simulink model "Gui"  (R2020b)
settings: Solver=VariableStepAuto  StartTime=0.0  StopTime=inf  RelTol=1e-3
libraries: simulink x7
settings Model: Creator=Axela  LastModifiedBy=MSI PC

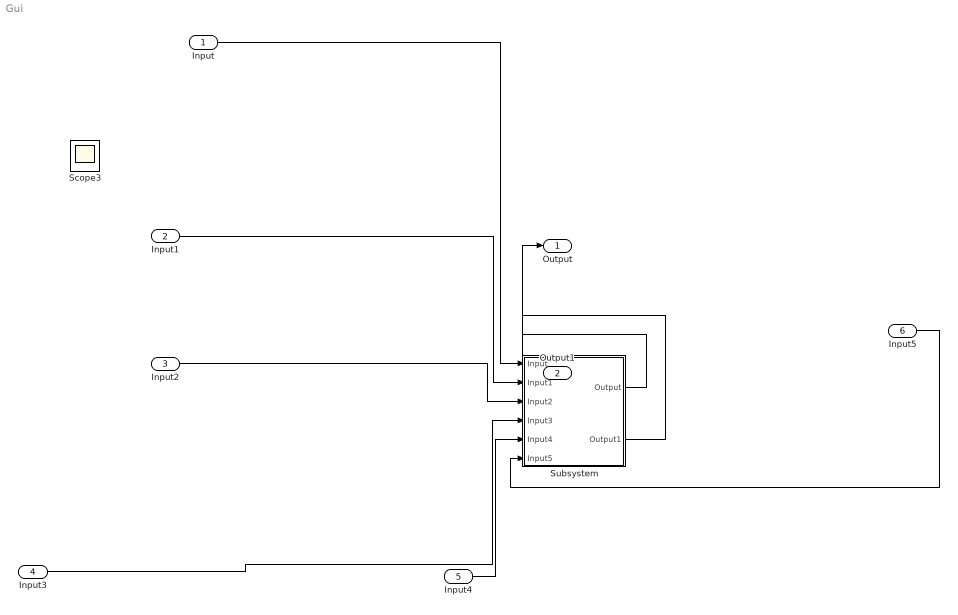
== system Gui ==
  Input : Inport
  Input1 : Inport  Port=2
  Input2 : Inport  Port=3
  Input3 : Inport  Port=4
  Input4 : Inport  Port=5
  Input5 : Inport  Port=6
  Subsystem : Subsystem
  Output : Outport
  Output1 : Outport  Port=2
  Scope3 : Scope
  wires:
  Input/1 -> Subsystem/1(Input)
  Input1/1 -> Subsystem/2(Input1)
  Input2/1 -> Subsystem/3(Input2)
  Input3/1 -> Subsystem/4(Input3)
  Input4/1 -> Subsystem/5(Input4)
  Input5/1 -> Subsystem/6(Input5)
  Subsystem/1(Output) -> Output/1
  Subsystem/2(Output1) -> Output1/1

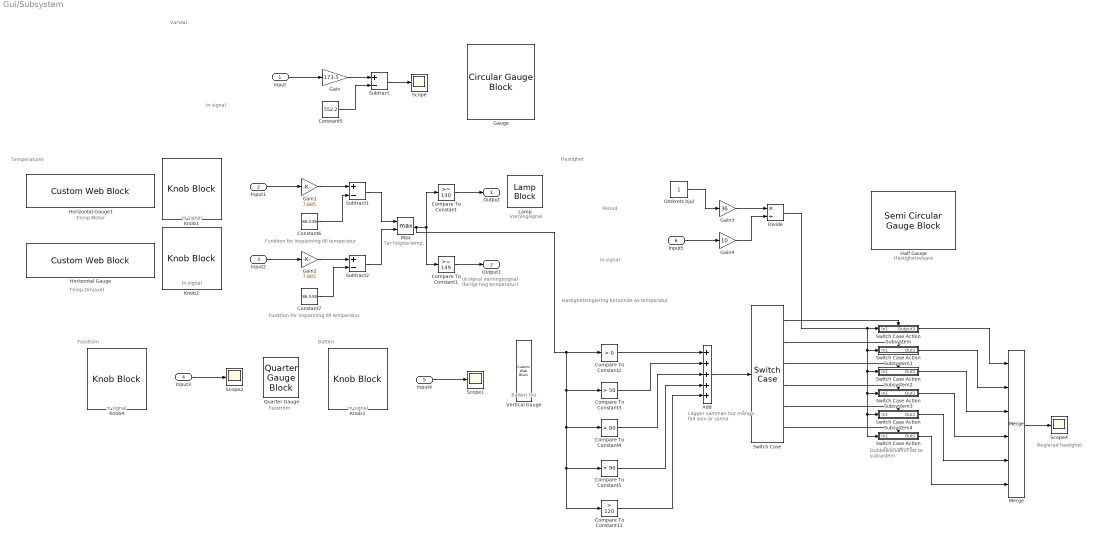
== system Gui/Subsystem ==
  note: in-signal
  note: Tar högsta temp.
  note: Funktion för inspänning till temperatur
  note: Temp.Drivaxel
  note: Temp.Motor
  note: Hastighetsvisare
  note: Reglerad hastighet
  note: Dubbelklicka för att se
      | subsystem
  note: Lägger samman
      | hur många fall
      | som är sanna
  note: Varningsignal
  note: ut-signal varningssignal
      | (farligt hög temperatur)
  note: Fasström
  note: Batteri (%)
  note: in-signal
  note: Hastighetsreglering beroende av temperatur
  note: Batteri
  note: Fasström
  note: Varvtal
  note: Temperaturer
  note: Hastighet
  note: Period
  note: in-signal
  note: in-signal
  note: in-signal
  note: in-signal
  note: Funktion för inspänning till temperatur
  Input : Inport
  Input1 : Inport  Port=2
  Input2 : Inport  Port=3
  Input3 : Inport  Port=4
  Input4 : Inport  Port=5
  Input5 : Inport  Port=6
  Add : Sum  Inputs=+++++
  Compare To Constant : simulink/Logic and Bit Operations/Compare To Constant  relop=>=  const=130  OutDataTypeStr=boolean
  Compare To Constant1 : simulink/Logic and Bit Operations/Compare To Constant  relop=>=  const=149  OutDataTypeStr=boolean
  Compare To Constant11 : simulink/Logic and Bit Operations/Compare To Constant  relop=>  const=120  OutDataTypeStr=boolean
  Compare To Constant2 : simulink/Logic and Bit Operations/Compare To Constant  relop=>  const=0  OutDataTypeStr=boolean
  Compare To Constant3 : simulink/Logic and Bit Operations/Compare To Constant  relop=>  const=50  OutDataTypeStr=boolean
  Compare To Constant4 : simulink/Logic and Bit Operations/Compare To Constant  relop=>  const=80  OutDataTypeStr=boolean
  Compare To Constant5 : simulink/Logic and Bit Operations/Compare To Constant  relop=>  const=90  OutDataTypeStr=boolean
  Constant5 : Constant  Value=552.2
  Constant6 : Constant  Value=86.538
  Constant7 : Constant  Value=86.538
  Divide : Product  Inputs=*/
  Gain : Gain  Gain=173.5
  Gain1 : Gain  Gain=7.885
  Gain2 : Gain  Gain=7.885
  Gain3 : Gain  Gain=36
  Gain4 : Gain  Gain=10
  Gauge : CircularGaugeBlock  LabelPosition=Hide
  Half Gauge : SemiCircularGaugeBlock  LabelPosition=Hide
  Horizontal Gauge : CustomWebBlock  LabelPosition=Hide  ShowInitialText=on  Configuration="{\"components\":[{\"name\":\"LinearScaleComponent\",\"settings\":{\"bounds\":{\"max\":100,\"min\":0,\"tickInterval\":\"auto\"},\"internalTickHeightScaleFactor\":0.5,\"labelColor\":[250,245,199],\"labelFont\":{\"font\":\"Arial\",\"fontSize\":12},\"labelTransparency\":1,\"needleImage\":{\"size\":[21,75],\"src\":\"data:image\\/svg+xml;base64,PHN2ZyB4bWxucz0iaHR0cDovL3d3dy53My5vcmcvMjAwMC9zdmciIHhtbG5zOnhsaW5rPSJodHRwOi8vd3d3LnczLm9yZy8xOTk5L3hsaW5rIiB2aWV3Qm94PSIwIDAgMjEgNzUiPjxkZWZzPjxzdHlsZT4uY2xzLTF7ZmlsbDpub25lO30uY2xzLTJ7aXNvbGF0aW9uOmlzb2xhdGU7fS5jbHMtM3tjbGlwLXBhdGg6dXJsKCNjbGlwLXBhdGgpO30uY2xzLTR7b3BhY2l0eTowLjM7bWl4LWJsZW5kLW1vZGU6bXVsdGlwbHk7fS5jbHMtNXtmaWxsOiNlYjI2Mjk7fTwvc3R5bGU+PGNsaXBQYXRoIGlkPSJjbGlwLXBhdGgiIHRyYW5zZm9y ...(+1928 chars)\",\"srcOrientation\":\"horizontal\"},\"needleOffset\":[0,0.01094391244870041],\"needleSize\":{\"height\":0.7589285714285714,\"width\":0.11960078534031414},\"position\":[0.06986607142857143,0.01995798319327731,0.9641544117647058,0.8],\"scaleColors\":[],\"scaleColorsSize\":0.2,\"showLabels\":1,\"showMinorTicks\":0,\"showSpanLine\":1,\"showTicks\":1,\"tickColor\":[250,245,200],\"tickTransparency\":1,\"valueBarColor\":[23,89,176],\"valueBarOffset\":0,\"valueBarSize\":0.23,\"valueBarTransparency\":1}},{\"name\":\"BackgroundImageComponent\",\"settings\":{\"image\":{\"size\":[380,101],\"src\":\"data:image\\/svg+xml;base64,PHN2ZyB4bWxucz0iaHR0cDovL3d3dy53My5vcmcvMjAwMC9zdmciIHZpZXdCb3g9IjAgMCAzODAgMTAxIj48ZGVmcz48c3R5bGU+LmNscy0xe2ZpbGw6IzAwMmI0Mjt9LmNscy0ye2ZpbGw6IzQyNzA4Mjt9LmNscy0ze2ZpbGw6IzdjYTBiMjt9PC9zdHlsZT48L2RlZnM+PHRpdGxlPmhvcml6b250YWxfZ2F1Z2VfIGJhY2tncm91bmQ8L3RpdGxlPjxnIGlkPSJMYXllcl8yIiBkYXRhLW5hbWU9IkxheWVyIDIiPjxnIGlkPSJMYXllcl8xLTIiIGRhdGEtbmFtZT0iTGF5ZXIgMSI+PHJlY3QgY2xhc3M9ImNscy0xIiB4PSIxMSIgeT0iMTEiIHdpZHRoPSIzNTgiIGhlaWdodD0iNzkiLz48cGF0aCBjbGFzcz0iY2xzLTIiIGQ9Ik04LDhWOTNIMzcyVjhaTTM2OSw5MEgxMVYxMUgzNjlaIi8+PHBhdGggY2xhc3M9ImNscy0zIiBkPSJNMCwwVjEwMUgzODBWMFpNMzcyLDkzSDhWOEgzNzJaIi8+PC9nPjwvZz48L3N2Zz4=\",\"srcOrientation\":\"horizontal\"},\"position\":[0,0,1,1],\"scaleMode\":\"0\"}},{\"name\":\"ForegroundImageComponent\",\"settings\":{\"image\":{\"size\":[0,0],\"src\":\"default\",\"srcOrientation\":[]},\"isForeground\":1,\"position\":[0,0,1,1],\"scaleMode\":\"0\"}}],\"settings\":{\"BindingType\":\"signal\",\"aspectRatio\":3.7721518987341773,\"fixedAspectRatio\":\"on\",\"orientation\":\"horizontal\"},\"type\":\"LinearGauge\"}"
  Horizontal Gauge1 : CustomWebBlock  LabelPosition=Hide  ShowInitialText=on  Configuration="{\"components\":[{\"name\":\"LinearScaleComponent\",\"settings\":{\"bounds\":{\"max\":100,\"min\":0,\"tickInterval\":\"auto\"},\"internalTickHeightScaleFactor\":0.5,\"labelColor\":[250,245,199],\"labelFont\":{\"font\":\"Arial\",\"fontSize\":12},\"labelTransparency\":1,\"needleImage\":{\"size\":[21,75],\"src\":\"data:image\\/svg+xml;base64,PHN2ZyB4bWxucz0iaHR0cDovL3d3dy53My5vcmcvMjAwMC9zdmciIHhtbG5zOnhsaW5rPSJodHRwOi8vd3d3LnczLm9yZy8xOTk5L3hsaW5rIiB2aWV3Qm94PSIwIDAgMjEgNzUiPjxkZWZzPjxzdHlsZT4uY2xzLTF7ZmlsbDpub25lO30uY2xzLTJ7aXNvbGF0aW9uOmlzb2xhdGU7fS5jbHMtM3tjbGlwLXBhdGg6dXJsKCNjbGlwLXBhdGgpO30uY2xzLTR7b3BhY2l0eTowLjM7bWl4LWJsZW5kLW1vZGU6bXVsdGlwbHk7fS5jbHMtNXtmaWxsOiNlYjI2Mjk7fTwvc3R5bGU+PGNsaXBQYXRoIGlkPSJjbGlwLXBhdGgiIHRyYW5zZm9y ...(+1928 chars)\",\"srcOrientation\":\"horizontal\"},\"needleOffset\":[0,0.01094391244870041],\"needleSize\":{\"height\":0.7589285714285714,\"width\":0.11960078534031414},\"position\":[0.06986607142857143,0.01995798319327731,0.9641544117647058,0.8],\"scaleColors\":[],\"scaleColorsSize\":0.2,\"showLabels\":1,\"showMinorTicks\":0,\"showSpanLine\":1,\"showTicks\":1,\"tickColor\":[250,245,200],\"tickTransparency\":1,\"valueBarColor\":[23,89,176],\"valueBarOffset\":0,\"valueBarSize\":0.23,\"valueBarTransparency\":1}},{\"name\":\"BackgroundImageComponent\",\"settings\":{\"image\":{\"size\":[380,101],\"src\":\"data:image\\/svg+xml;base64,PHN2ZyB4bWxucz0iaHR0cDovL3d3dy53My5vcmcvMjAwMC9zdmciIHZpZXdCb3g9IjAgMCAzODAgMTAxIj48ZGVmcz48c3R5bGU+LmNscy0xe2ZpbGw6IzAwMmI0Mjt9LmNscy0ye2ZpbGw6IzQyNzA4Mjt9LmNscy0ze2ZpbGw6IzdjYTBiMjt9PC9zdHlsZT48L2RlZnM+PHRpdGxlPmhvcml6b250YWxfZ2F1Z2VfIGJhY2tncm91bmQ8L3RpdGxlPjxnIGlkPSJMYXllcl8yIiBkYXRhLW5hbWU9IkxheWVyIDIiPjxnIGlkPSJMYXllcl8xLTIiIGRhdGEtbmFtZT0iTGF5ZXIgMSI+PHJlY3QgY2xhc3M9ImNscy0xIiB4PSIxMSIgeT0iMTEiIHdpZHRoPSIzNTgiIGhlaWdodD0iNzkiLz48cGF0aCBjbGFzcz0iY2xzLTIiIGQ9Ik04LDhWOTNIMzcyVjhaTTM2OSw5MEgxMVYxMUgzNjlaIi8+PHBhdGggY2xhc3M9ImNscy0zIiBkPSJNMCwwVjEwMUgzODBWMFpNMzcyLDkzSDhWOEgzNzJaIi8+PC9nPjwvZz48L3N2Zz4=\",\"srcOrientation\":\"horizontal\"},\"position\":[0,0,1,1],\"scaleMode\":\"0\"}},{\"name\":\"ForegroundImageComponent\",\"settings\":{\"image\":{\"size\":[0,0],\"src\":\"default\",\"srcOrientation\":[]},\"isForeground\":1,\"position\":[0,0,1,1],\"scaleMode\":\"0\"}}],\"settings\":{\"BindingType\":\"signal\",\"aspectRatio\":3.7721518987341773,\"fixedAspectRatio\":\"on\",\"orientation\":\"horizontal\"},\"type\":\"LinearGauge\"}"
  Knob1 : KnobBlock  LabelPosition=Hide  ScaleMin=4  ScaleMax=30
  Knob2 : KnobBlock  LabelPosition=Hide  ScaleMin=4  ScaleMax=30
  Knob3 : KnobBlock  LabelPosition=Hide
  Knob4 : KnobBlock  LabelPosition=Hide
  Lamp : LampBlock  LabelPosition=Hide
  Max : MinMax  Function=max  Inputs=2
  Merge : Merge  Inputs=6
  Omkrets hjul : Constant
  Quarter Gauge : QuarterGaugeBlock  LabelPosition=Hide
  Scope{,1..2,4} (4 alike) : Scope
  Subtract : Sum  Inputs=+-
  Subtract1 : Sum  Inputs=+-
  Subtract2 : Sum  Inputs=+-
  Switch Case : SwitchCase  CaseConditions={1,2,3,4,5}
  Switch Case Action Subsystem : Subsystem  TreatAsAtomicUnit=on
  Switch Case Action Subsystem1 : Subsystem  TreatAsAtomicUnit=on
  Switch Case Action Subsystem2 : Subsystem  TreatAsAtomicUnit=on
  Switch Case Action Subsystem3 : Subsystem  TreatAsAtomicUnit=on
  Switch Case Action Subsystem4 : Subsystem  TreatAsAtomicUnit=on
  Switch Case Action Subsystem5 : Subsystem  TreatAsAtomicUnit=on
  Vertical Gauge : CustomWebBlock  LabelPosition=Hide  ShowInitialText=on  Configuration="{\"components\":[{\"name\":\"LinearScaleComponent\",\"settings\":{\"bounds\":{\"max\":100,\"min\":0,\"tickInterval\":\"auto\"},\"internalTickHeightScaleFactor\":0.5,\"labelColor\":[250,245,199],\"labelFont\":{\"font\":\"Arial\",\"fontSize\":12},\"labelTransparency\":1,\"needleImage\":{\"size\":[21,75],\"src\":\"data:image\\/svg+xml;base64,PHN2ZyB4bWxucz0iaHR0cDovL3d3dy53My5vcmcvMjAwMC9zdmciIHhtbG5zOnhsaW5rPSJodHRwOi8vd3d3LnczLm9yZy8xOTk5L3hsaW5rIiB2aWV3Qm94PSIwIDAgMjEgNzUiPjxkZWZzPjxzdHlsZT4uY2xzLTF7ZmlsbDpub25lO30uY2xzLTJ7aXNvbGF0aW9uOmlzb2xhdGU7fS5jbHMtM3tjbGlwLXBhdGg6dXJsKCNjbGlwLXBhdGgpO30uY2xzLTR7b3BhY2l0eTowLjM7bWl4LWJsZW5kLW1vZGU6bXVsdGlwbHk7fS5jbHMtNXtmaWxsOiNlYjI2Mjk7fTwvc3R5bGU+PGNsaXBQYXRoIGlkPSJjbGlwLXBhdGgiIHRyYW5zZm9y ...(+1928 chars)\",\"srcOrientation\":\"horizontal\"},\"needleOffset\":[-0.01094391244870041,0],\"needleSize\":{\"height\":0.11960078534031414,\"width\":0.7589285714285714},\"position\":[0.015887605042016806,0.06986607142857143,0.8,0.9641544117647058],\"scaleColors\":[],\"scaleColorsSize\":0.2,\"showLabels\":1,\"showMinorTicks\":0,\"showSpanLine\":1,\"showTicks\":1,\"tickColor\":[250,245,200],\"tickTransparency\":1,\"valueBarColor\":[23,89,176],\"valueBarOffset\":0,\"valueBarSize\":0.23,\"valueBarTransparency\":1}},{\"name\":\"BackgroundImageComponent\",\"settings\":{\"image\":{\"size\":[101,380],\"src\":\"data:image\\/svg+xml;base64,PHN2ZyB4bWxucz0iaHR0cDovL3d3dy53My5vcmcvMjAwMC9zdmciIHZpZXdCb3g9IjAgMCAxMDEgMzgwIj48ZGVmcz48c3R5bGU+LmNscy0xe2ZpbGw6IzAwMmI0Mjt9LmNscy0ye2ZpbGw6IzQyNzA4Mjt9LmNscy0ze2ZpbGw6IzdjYTBiMjt9PC9zdHlsZT48L2RlZnM+PHRpdGxlPnZlcnRpY2FsX2dhdWdlX2JhY2tncm91bmRfMTwvdGl0bGU+PGcgaWQ9IkxheWVyXzIiIGRhdGEtbmFtZT0iTGF5ZXIgMiI+PGcgaWQ9IkxheWVyXzEtMiIgZGF0YS1uYW1lPSJMYXllciAxIj48cmVjdCBjbGFzcz0iY2xzLTEiIHg9IjExIiB5PSIxMSIgd2lkdGg9Ijc5IiBoZWlnaHQ9IjM1OCIvPjxwYXRoIGNsYXNzPSJjbHMtMiIgZD0iTTkzLDhIOFYzNzJIOTNaTTExLDM2OVYxMUg5MFYzNjlaIi8+PHBhdGggY2xhc3M9ImNscy0zIiBkPSJNMTAxLDBIMFYzODBIMTAxWk04LDM3MlY4SDkzVjM3MloiLz48L2c+PC9nPjwvc3ZnPg==\",\"srcOrientation\":\"vertical\"},\"position\":[0,0,1,1],\"scaleMode\":\"0\"}},{\"name\":\"ForegroundImageComponent\",\"settings\":{\"image\":{\"size\":[0,0],\"src\":\"default\",\"srcOrientation\":[]},\"isForeground\":1,\"position\":[0,0,1,1],\"scaleMode\":\"0\"}}],\"settings\":{\"BindingType\":\"signal\",\"aspectRatio\":0.2647058823529412,\"fixedAspectRatio\":\"on\",\"orientation\":\"vertical\"},\"type\":\"LinearGauge\"}"
  Output : Outport
  Output1 : Outport  Port=2
  wires:
  Constant5/1 -> Subtract/2
  Switch Case/4 -> Switch Case Action Subsystem3/Action
  Input5/1 -> Gain4/1
  Subtract/1 -> Scope/1
  Input1/1 -> Gain1/1
  Merge/1 -> Scope4/1
  Compare To Constant11/1 -> Add/5
  Constant6/1 -> Subtract1/2
  Max/1 -> Compare To Constant/1, Compare To Constant1/1, Compare To Constant2/1, Compare To Constant11/1, Compare To Constant5/1, Compare To Constant4/1, Compare To Constant3/1
  Gain1/1 -> Subtract1/1
  Input3/1 -> Scope2/1
  Switch Case/5 -> Switch Case Action Subsystem4/Action
  Gain4/1 -> Divide/2
  Constant7/1 -> Subtract2/2
  Divide/1 -> Switch Case Action Subsystem/1(In1), Switch Case Action Subsystem5/1(In1), Switch Case Action Subsystem4/1(In1), Switch Case Action Subsystem3/1(In1), Switch Case Action Subsystem2/1(In1), Switch Case Action Subsystem1/1(In1)
  Gain2/1 -> Subtract2/1
  Compare To Constant/1 -> Output/1
  Gain3/1 -> Divide/1
  Compare To Constant2/1 -> Add/1
  Input2/1 -> Gain2/1
  Gain/1 -> Subtract/1
  Switch Case Action Subsystem/1(Output3) -> Merge/1
  Subtract2/1 -> Max/2
  Switch Case Action Subsystem5/1(Out1) -> Merge/6
  Subtract1/1 -> Max/1
  Omkrets hjul/1 -> Gain3/1
  Add/1 -> Switch Case/1
  Compare To Constant3/1 -> Add/2
  Compare To Constant5/1 -> Add/4
  Compare To Constant1/1 -> Output1/1
  Compare To Constant4/1 -> Add/3
  Switch Case/2 -> Switch Case Action Subsystem1/Action
  Switch Case Action Subsystem3/1(Out1) -> Merge/4
  Switch Case/6 -> Switch Case Action Subsystem5/Action
  Switch Case Action Subsystem4/1(Out1) -> Merge/5
  Switch Case/3 -> Switch Case Action Subsystem2/Action
  Switch Case Action Subsystem1/1(Out1) -> Merge/2
  Switch Case/1 -> Switch Case Action Subsystem/Action
  Switch Case Action Subsystem2/1(Out1) -> Merge/3
  Input4/1 -> Scope1/1
  Input/1 -> Gain/1

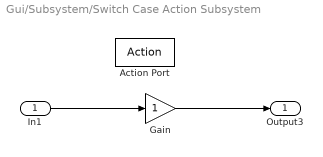
== system Gui/Subsystem/Switch Case Action Subsystem ==
  In1 : Inport
  Action Port : ActionPort  ActionPortLabel=case [ 1 ]:
  Gain : Gain
  Output3 : Outport
  wires:
  In1/1 -> Gain/1
  Gain/1 -> Output3/1

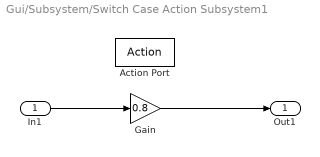
== system Gui/Subsystem/Switch Case Action Subsystem1 ==
  In1 : Inport
  Action Port : ActionPort  ActionPortLabel=case [ 2 ]:
  Gain : Gain  Gain=0.8
  Out1 : Outport
  wires:
  In1/1 -> Gain/1
  Gain/1 -> Out1/1

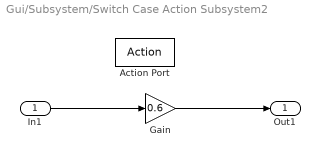
== system Gui/Subsystem/Switch Case Action Subsystem2 ==
  In1 : Inport
  Action Port : ActionPort  ActionPortLabel=case [ 3 ]:
  Gain : Gain  Gain=0.6
  Out1 : Outport
  wires:
  In1/1 -> Gain/1
  Gain/1 -> Out1/1

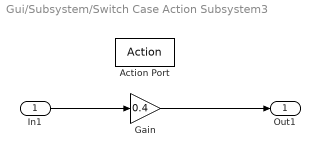
== system Gui/Subsystem/Switch Case Action Subsystem3 ==
  In1 : Inport
  Action Port : ActionPort  ActionPortLabel=case [ 4 ]:
  Gain : Gain  Gain=0.4
  Out1 : Outport
  wires:
  In1/1 -> Gain/1
  Gain/1 -> Out1/1

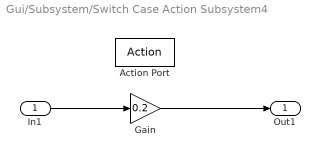
== system Gui/Subsystem/Switch Case Action Subsystem4 ==
  In1 : Inport
  Action Port : ActionPort  ActionPortLabel=case [ 5 ]:
  Gain : Gain  Gain=0.2
  Out1 : Outport
  wires:
  In1/1 -> Gain/1
  Gain/1 -> Out1/1

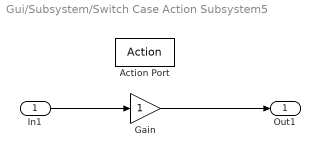
== system Gui/Subsystem/Switch Case Action Subsystem5 ==
  In1 : Inport
  Action Port : ActionPort  ActionPortLabel=default:
  Gain : Gain
  Out1 : Outport
  wires:
  In1/1 -> Gain/1
  Gain/1 -> Out1/1
